simulink model "ep6_1_2"  (R2018a)
settings: Solver=VariableStepAuto  StartTime=0.0  StopTime=20  MaxStep=0.001  RelTol=1e-3
settings Model: Creator=zheny  LastModifiedBy=zheny

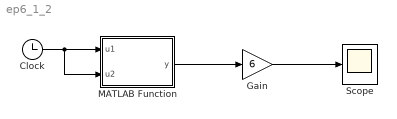
== system ep6_1_2 ==
  Clock : Clock
  Gain : Gain  Gain=6
  MATLAB Function : MATLAB Function  TreatAsAtomicUnit=on
  Scope : Scope
  wires:
  Gain/1 -> Scope/1
  Clock/1 -> MATLAB Function/2(u2), MATLAB Function/1(u1)
  MATLAB Function/1(y) -> Gain/1

== matlab function ep6_1_2/MATLAB Function ==
  data: u1 input; y output; u2 input
function y = fcn(u1, u2)

y = sin(u1) + cos(u2);
